simulink model "Assignment_2__Task2"  (R2019b)
settings: Solver=VariableStepAuto  StartTime=0.0  StopTime=10.0  RelTol=1e-3
values from neighbouring files (symbols this model uses):
  A = [0 0 1 0; 0 0 0 1; 0 a32 a33 a34; 0 a42 a43 a44]    [Assignment_2_Task 1.m]
  B = [0; 0; 1/mc; 1/(L*mc)]    [Assignment_2_Task 1.m]
  C = [0 1 0 0]    [Assignment_2_Task 1.m]
undefined symbols (not defined in the file or in its folder): x0
settings Model: Creator=Vishrant  LastModifiedBy=Vishrant

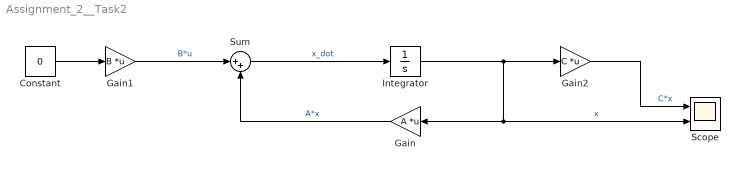
== system Assignment_2__Task2 ==
  Constant : Constant  Value=0
  Gain : Gain  Gain=A  Multiplication=Matrix(K*u)
  Gain1 : Gain  Gain=B  Multiplication=Matrix(K*u)
  Gain2 : Gain  Gain=C  Multiplication=Matrix(K*u)
  Integrator : Integrator  InitialCondition=x0
  Scope : Scope  NumInputPorts=2
  Sum : Sum  Inputs=|++
  wires:
  Integrator/1 -> Gain2/1, Gain/1, Scope/2  "x"
  Sum/1 -> Integrator/1  "x_dot"
  Gain1/1 -> Sum/1  "B*u"
  Gain/1 -> Sum/2  "A*x"
  Gain2/1 -> Scope/1  "C*x"
  Constant/1 -> Gain1/1
